simulink model "BlockDiagram"  (R2024b)
settings: Solver=VariableStepAuto  StartTime=0.0  StopTime=10.0  RelTol=1e-3
model workspace (MAT data in the model file):
  G1 = 1
  G2 = 1
  H = 1
  IRdata = 1
  Kd = 1
  Kff = 1
  Ki = 1
  Kp = 1
  Kw = 1
  PWMstartL = 1
  r = 0
  vref = 1
undefined symbols (not defined in the file): PWMstartR
settings Model: Creator=caidenbonney  LastModifiedBy=Caide

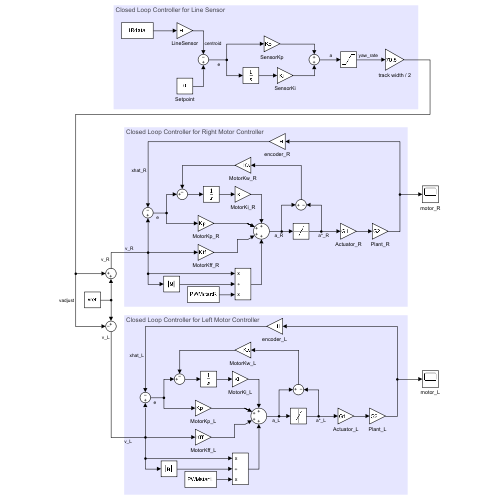
[thumbnail: Simulink's stored preview of the top-level diagram]
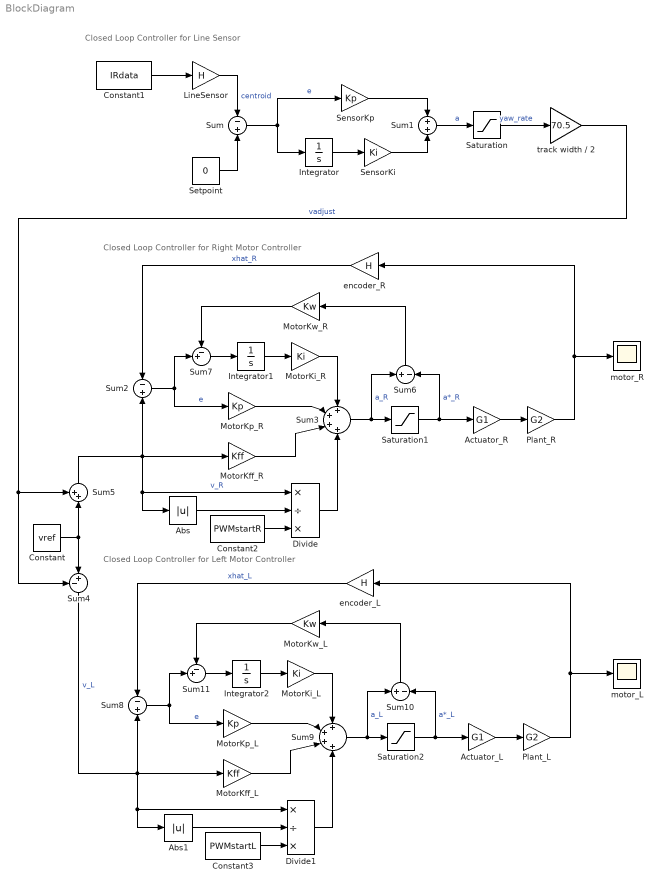
== system BlockDiagram ==
  note: Closed Loop Controller for Right Motor Controller
  note: Closed Loop Controller for Line Sensor
  note: Closed Loop Controller for Left Motor Controller
  Abs : Abs  SaturateOnIntegerOverflow=off
  Abs1 : Abs  SaturateOnIntegerOverflow=off
  Actuator_L : Gain  Gain=G1
  Actuator_R : Gain  Gain=G1
  Constant : Constant  Value=vref
  Constant1 : Constant  Value=IRdata
  Constant2 : Constant  Value=PWMstartR
  Constant3 : Constant  Value=PWMstartL
  Divide : Product  Inputs=*/*
  Divide1 : Product  Inputs=*/*
  Integrator : Integrator
  Integrator1 : Integrator
  Integrator2 : Integrator
  LineSensor : Gain  Gain=H
  MotorKff_L : Gain  Gain=Kff
  MotorKff_R : Gain  Gain=Kff
  MotorKi_L : Gain  Gain=Ki
  MotorKi_R : Gain  Gain=Ki
  MotorKp_L : Gain  Gain=Kp
  MotorKp_R : Gain  Gain=Kp
  MotorKw_L : Gain  Gain=Kw
  MotorKw_R : Gain  Gain=Kw
  Plant_L : Gain  Gain=G2
  Plant_R : Gain  Gain=G2
  Saturation : Saturate
  Saturation1 : Saturate
  Saturation2 : Saturate
  SensorKi : Gain  Gain=Ki
  SensorKp : Gain  Gain=Kp
  Setpoint : Constant  Value=0
  Sum : Sum  Inputs=-|+
  Sum1 : Sum
  Sum10 : Sum  Inputs=+-
  Sum11 : Sum  Inputs=-+|
  Sum2 : Sum  Inputs=-|+
  Sum3 : Sum  Inputs=++++
  Sum4 : Sum  Inputs=-+|
  Sum5 : Sum  Inputs=++|
  Sum6 : Sum  Inputs=+-
  Sum7 : Sum  Inputs=-+|
  Sum8 : Sum  Inputs=-|+
  Sum9 : Sum  Inputs=++++
  encoder_L : Gain  Gain=H
  encoder_R : Gain  Gain=H
  motor_L : Scope
  motor_R : Scope
  track width / 2 : Gain  Gain=70.5
  wires:
  Setpoint/1 -> Sum/2
  LineSensor/1 -> Sum/1  "centroid"
  Sum/1 -> SensorKp/1, Integrator/1  "e"
  Integrator/1 -> SensorKi/1
  SensorKp/1 -> Sum1/1
  SensorKi/1 -> Sum1/2
  Sum1/1 -> Saturation/1  "a"
  Saturation/1 -> track width / 2/1  "yaw_rate"
  Plant_R/1 -> encoder_R/1, motor_R/1
  Actuator_R/1 -> Plant_R/1
  Saturation1/1 -> Sum6/2, Actuator_R/1  "a*_R"
  Sum3/1 -> Saturation1/1, Sum6/1  "a_R"
  MotorKi_R/1 -> Sum3/1
  MotorKp_R/1 -> Sum3/2
  Integrator1/1 -> MotorKi_R/1
  Sum2/1 -> Sum7/2, MotorKp_R/1  "e"
  encoder_R/1 -> Sum2/1  "xhat_R"
  track width / 2/1 -> Sum4/1, Sum5/1  "vadjust"
  Constant1/1 -> LineSensor/1
  Constant/1 -> Sum4/2, Sum5/2
  Sum5/1 -> MotorKff_R/1, Sum2/2, Divide/1, Abs/1  "v_R"
  Sum4/1 -> Sum8/2, Abs1/1, Divide1/1, MotorKff_L/1  "v_L"
  MotorKff_R/1 -> Sum3/3
  Constant2/1 -> Divide/3
  Abs/1 -> Divide/2
  Divide/1 -> Sum3/4
  Sum6/1 -> MotorKw_R/1
  MotorKw_R/1 -> Sum7/1
  Sum7/1 -> Integrator1/1
  Sum11/1 -> Integrator2/1
  MotorKw_L/1 -> Sum11/1
  Sum10/1 -> MotorKw_L/1
  Divide1/1 -> Sum9/4
  Abs1/1 -> Divide1/2
  Constant3/1 -> Divide1/3
  MotorKff_L/1 -> Sum9/3
  encoder_L/1 -> Sum8/1  "xhat_L"
  Sum8/1 -> MotorKp_L/1, Sum11/2  "e"
  Integrator2/1 -> MotorKi_L/1
  MotorKp_L/1 -> Sum9/2
  MotorKi_L/1 -> Sum9/1
  Sum9/1 -> Sum10/1, Saturation2/1  "a_L"
  Saturation2/1 -> Actuator_L/1, Sum10/2  "a*_L"
  Actuator_L/1 -> Plant_L/1
  Plant_L/1 -> encoder_L/1, motor_L/1
